simulink model "cic_dezim_interp1"  (Simulink 7.8)
settings: Solver=FixedStepDiscrete  SolverMode=SingleTasking  StartTime=0.0  StopTime=1  RelTol=1e-3
undefined symbols (not defined in the file or in its folder): get
libraries: dspsnks4 x3, dspmlti4 x2
settings Model: Creator=svenhoffmann  LastModifiedBy=josef  ExtModeAutoUpdateStatusClock=off
settings OptimizationCC: InlineInvariantSignals=on  InitFltsAndDblsToZero=on
settings DebuggingCC: SaveWithParameterizedLinksMsg=none  SignalResolutionControl=TryResolveAllWithWarning  MultiTaskDSMMsg=warning  MultiTaskCondExecSysMsg=none  StrictBusMsg=None
settings RTWCC: IncludeERTFirstTime=on
settings GRTTargetCC: TargetFcnLib=ansi_tfl_tmw.mat

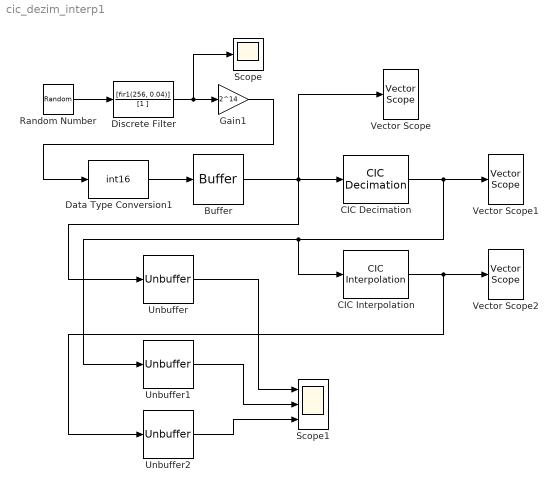
== system cic_dezim_interp1 ==
  Buffer : Buffer  N=100
  CIC Decimation : dspmlti4/CIC Decimation  filtFrom=Dialog  filtobj=Hm_decim  ftype=Decimator  R=5  M=1  N=5  filterInternals=Full precision  BPS=[28 28 28 28 28 28 28 28 28 16]  FLPS=0  outputWordLength=32  outputFracLength=0  launchFVT=off  framing=Maintain input frame rate  RateOptions=Inherit from input (this choice will be removed - see release notes)
  CIC Interpolation : dspmlti4/CIC Interpolation  filtFrom=Dialog  filtobj=Hm_interp  ftype=Interpolator  R=5  M=1  N=5  filterInternals=Full precision  BPS=[17 18 19 20 21 21 22 23 24 26]  FLPS=0  outputWordLength=32  outputFracLength=0  launchFVT=off  framing=Maintain input frame rate  InputProcessing=Inherited (this choice will be removed - see release notes)
  Data Type Conversion1 : DataTypeConversion  OutDataTypeStr=int16
  Discrete Filter : DiscreteFilter  Numerator=[fir1(256, 0.04)]  Denominator=[1 ]
  Gain1 : Gain  Gain=2^14  OutDataTypeStr=Inherit: Same as input
  Random Number : RandomNumber  SampleTime=1/10000
  Scope : Scope
  Scope1 : Scope  NumInputPorts=3
      settings: TimeRange=0.1  YMin=-10000~-3e+07~-2e+10  YMax=12500~4e+07~2.5e+10
  Unbuffer : Unbuffer
  Unbuffer1 : Unbuffer
  Unbuffer2 : Unbuffer
  Vector Scope : dspsnks4/Vector Scope  ScopeProperties=on  Domain=Time  HorizSpan=10  DisplayProperties=off  AxisGrid=on  Memory=off  FrameNumber=on  AxisLegend=off  AxisZoom=off  OpenScopeAtSimStart=on  OpenScopeImmediately=off  FigPos=get(0,'defaultfigureposition')  AxisProperties=off  XUnits=Hertz  XRange=[0...Fs/2]  InheritXIncr=on  XIncr=1  XLabel=Time  XLimit=Auto  XMin=0  XMax=1  XStart=0  YUnits=dB  YLabel=Amplitude  LineProperties=off  XAxisParamsVer=6.8
      settings: YMin=-7791  YMax=6293.7
  Vector Scope1 : dspsnks4/Vector Scope  ScopeProperties=on  Domain=Time  HorizSpan=10  DisplayProperties=off  AxisGrid=on  Memory=off  FrameNumber=on  AxisLegend=off  AxisZoom=off  OpenScopeAtSimStart=on  OpenScopeImmediately=off  FigPos=get(0,'defaultfigureposition')  AxisProperties=off  XUnits=Hertz  XRange=[0...Fs/2]  InheritXIncr=on  XIncr=1  XLabel=Time  XLimit=Auto  XMin=0  XMax=1  XStart=0  YUnits=dB  YLabel=Amplitude  LineProperties=off  XAxisParamsVer=6.8
      settings: YMin=-23327539.2  YMax=18785894.4
  Vector Scope2 : dspsnks4/Vector Scope  ScopeProperties=on  Domain=Time  HorizSpan=10  DisplayProperties=off  AxisGrid=on  Memory=off  FrameNumber=on  AxisLegend=off  AxisZoom=off  OpenScopeAtSimStart=on  OpenScopeImmediately=off  FigPos=get(0,'defaultfigureposition')  AxisProperties=off  XUnits=Hertz  XRange=[0...Fs/2]  InheritXIncr=on  XIncr=1  XLabel=Time  XLimit=Auto  XMin=0  XMax=1  XStart=0  YUnits=dB  YLabel=Amplitude  LineProperties=off  XAxisParamsVer=6.8
      settings: YMin=-14385659904  YMax=11427053568
  wires:
  Buffer/1 -> CIC Decimation/1, Vector Scope/1, Unbuffer/1
  CIC Decimation/1 -> Vector Scope1/1, CIC Interpolation/1, Unbuffer1/1
  Random Number/1 -> Discrete Filter/1
  Discrete Filter/1 -> Gain1/1, Scope/1
  Gain1/1 -> Data Type Conversion1/1
  CIC Interpolation/1 -> Vector Scope2/1, Unbuffer2/1
  Unbuffer/1 -> Scope1/1
  Unbuffer1/1 -> Scope1/2
  Unbuffer2/1 -> Scope1/3
  Data Type Conversion1/1 -> Buffer/1
